simulink model "Model7"  (R2022b)
settings: Solver=VariableStepAuto  StartTime=0.0  StopTime=10.0  RelTol=1e-3
model workspace (MAT data in the model file):
  Freq = Simulink.Parameter
  Freq.Value = 2000000
  Freq.DataType = 'auto'
  Freq.Complexity = 'real'
  Freq.Dimensions = [1 1]
  Freq2 = Simulink.Parameter
  Freq2.Value = 6000000
  Freq2.DataType = 'auto'
  Freq2.Complexity = 'real'
  Freq2.Dimensions = [1 1]
  Freq3 = Simulink.Parameter
  Freq3.Value = 3000000
  Freq3.DataType = 'auto'
  Freq3.Complexity = 'real'
  Freq3.Dimensions = [1 1]
  Freq4 = Simulink.Parameter
  Freq4.Value = 10000000
  Freq4.DataType = 'auto'
  Freq4.Complexity = 'real'
  Freq4.Dimensions = [1 1]
  fsr = 20
libraries: commdigbbndam3 x5, commrandsrc3 x4, dspfdesign x2, commchan3 x1, commsink2 x1, commutil2 x1, simulink x1
settings Model: Creator=Ceribro  LastModifiedBy=Ceribro

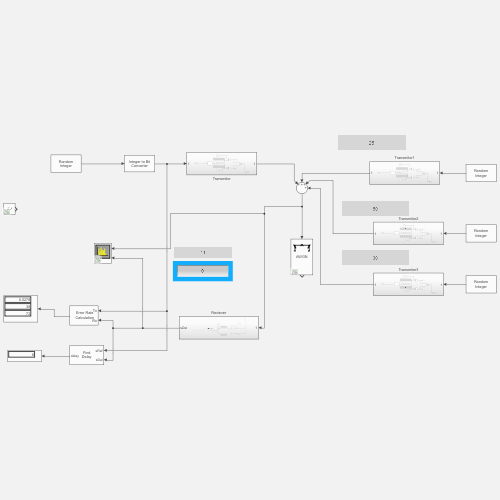
[thumbnail: Simulink's stored preview of the top-level diagram]
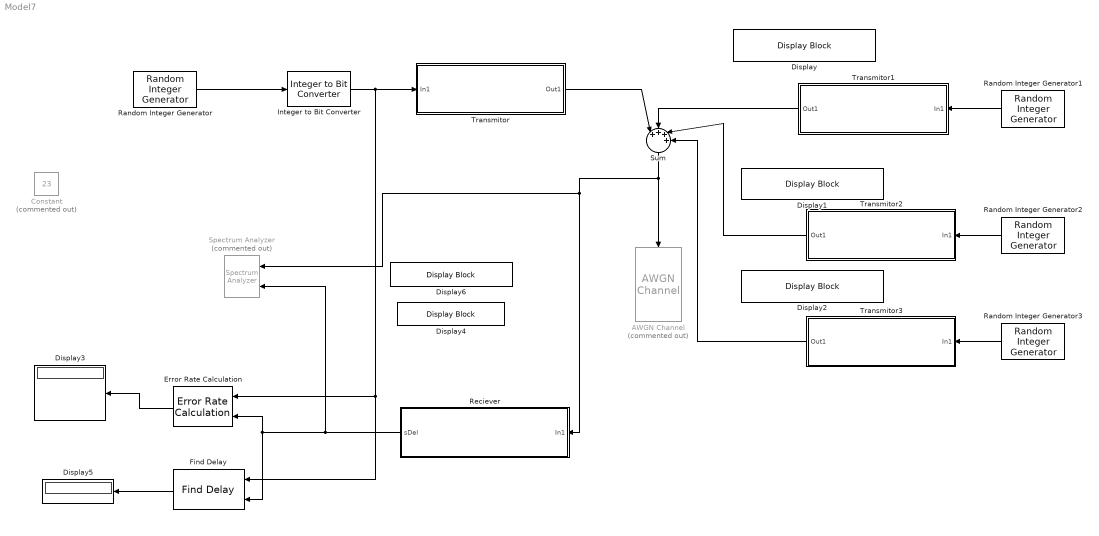
== system Model7 ==
  AWGN Channel : commchan3/AWGN Channel  Commented=on  InputProcessing=Columns as channels (frame based)  seed=67  noiseMode="Signal to noise ratio  (SNR)"  EbNodB=10  EsNodB=10  SNRdB=-10  bitsPerSym=1  Ps=1  Tsym=1  variance=1
  Constant : Constant  Commented=on  Value=23  SampleTime=0.01
  Display{,1..2,4,6} (5 alike) : DisplayBlock  LabelPosition=Hide  Transparency=1
  Display3 : Display
  Display5 : Display
  Error Rate Calculation : commsink2/Error Rate Calculation  N=0  st_delay=0  cp_mode=Entire frame  subframe=[]  PMode=Port  WsName=ErrorVec  RsMode2=off  stop=off  numErr=100  maxBits=1e6
      settings: LibrarySourceBlock=|
      | commhdlsink/Error Rate
      | Calculation
  Find Delay : commutil2/Find Delay  corrLength=10  chgSigOP=off  stopUpdate=off  numConstDelay=3
  Integer to Bit Converter : simulink/Logic and Bit Operations/Integer to Bit Converter  nbits=6  signedInputValues=Unsigned  bitOrder=MSB first  outDtype=Inherit via internal rule
  Random Integer Generator{,1..3} (4 alike) : commrandsrc3/Random Integer Generator  SetSize=64  SeedSource=Auto  Seed=0  SampleTime=0.1  SamplesPerFrame=1  OutputDataType=double  SimulateUsing=Interpreted execution
  Reciever : Subsystem
  Spectrum Analyzer : SpectrumAnalyzer  Commented=on  NumInputPorts=2
  Sum : Sum  Inputs=|++++
  Transmitor : Subsystem
  Transmitor1 : Subsystem
  Transmitor2 : Subsystem
  Transmitor3 : Subsystem
  wires:
  Transmitor/1(Out1) -> Sum/1
  Random Integer Generator/1 -> Integer to Bit Converter/1
  Random Integer Generator1/1 -> Transmitor1/1(In1)
  Sum/1 -> Spectrum Analyzer/1, Reciever/1(In1), AWGN Channel/1
  Transmitor1/1(Out1) -> Sum/2
  Transmitor2/1(Out1) -> Sum/3
  Random Integer Generator2/1 -> Transmitor2/1(In1)
  Random Integer Generator3/1 -> Transmitor3/1(In1)
  Transmitor3/1(Out1) -> Sum/4
  Find Delay/1 -> Display5/1
  Error Rate Calculation/1 -> Display3/1
  Reciever/1(sDel) -> Error Rate Calculation/2, Find Delay/2, Spectrum Analyzer/2
  Integer to Bit Converter/1 -> Find Delay/1, Error Rate Calculation/1, Transmitor/1(In1)

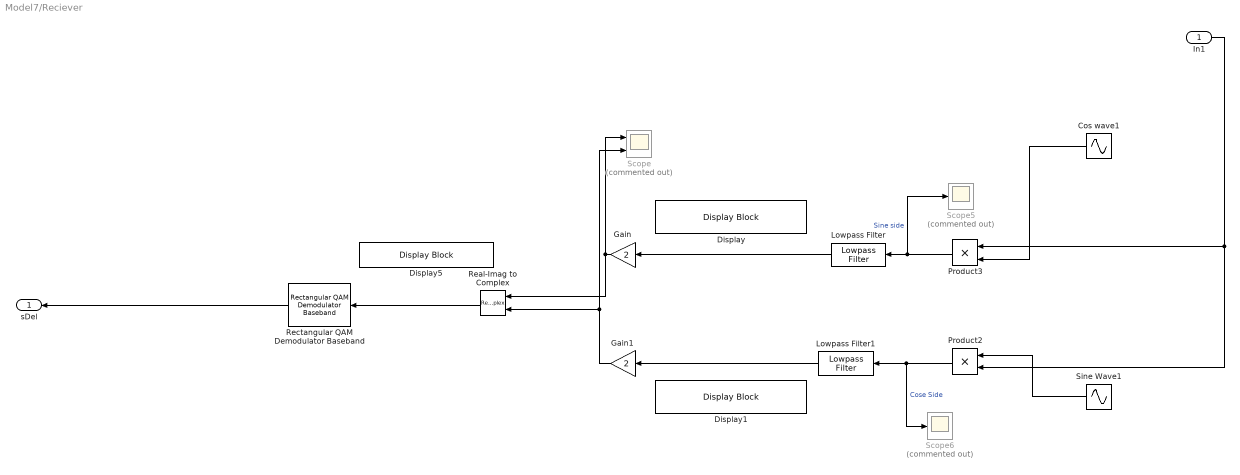
== system Model7/Reciever ==
  In1 : Inport
  Cos wave1 : Sin  Frequency=2*pi*Freq  Phase=pi/2  SampleTime=1/44100  VectorParams1D=off
  Display : DisplayBlock  LabelPosition=Hide  Transparency=1
  Display1 : DisplayBlock  LabelPosition=Hide  Transparency=1
  Display5 : DisplayBlock  LabelPosition=Hide  Transparency=1
  Gain : Gain  Gain=2
  Gain1 : Gain  Gain=2
  Lowpass Filter : dspfdesign/Lowpass Filter  FilterType=FIR  DesignForMinimumOrder=on  FilterOrder=50  PassbandFrequency=0.5e3  StopbandFrequency=1e3  PassbandRipple=0.1  StopbandAttenuation=80  InheritSampleRate=off  SampleRate=44100  SimulateUsing=Interpreted execution  roundingMode=Floor  coeffsDataTypeStr=fixdt(1,16)
  Lowpass Filter1 : dspfdesign/Lowpass Filter  FilterType=FIR  DesignForMinimumOrder=on  FilterOrder=50  PassbandFrequency=0.5e3  StopbandFrequency=1e3  PassbandRipple=0.1  StopbandAttenuation=80  InheritSampleRate=off  SampleRate=44100  SimulateUsing=Interpreted execution  roundingMode=Floor  coeffsDataTypeStr=fixdt(1,16)
  Product2 : Product
  Product3 : Product
  Real-Imag to Complex : RealImagToComplex
  Rectangular QAM Demodulator Baseband : commdigbbndam3/Rectangular QAM Demodulator Baseband  M=64  OutType=Bit  DecType=Hard decision  VarSource=Dialog  Variance=1  Dec=Binary  Mapping=[0:15]  PowType=Min. distance between symbols  MinDist=2  AvgPow=1  PeakPow=1  Ph=0  outDtype1=Inherit via internal rule  outDtype2=Inherit via internal rule  derotateFactorWordLen=16  derotateFactorDataTypeStr=Inherit: Same word length as input  derotateFactorLastDataTypeStr=Inherit: Same word length as input  denormFactorWordLen=16  denormFactorDataTypeStr=Inherit: Same word length as input  denormFactorLastDataTypeStr=Inherit: Same word length as input  prodOutWordLen=32  prodOutOverflowMode=Wrap  prodOutRoundingMode=Floor  prodOutOvFlMode=off  prodOutOvFlModeLastStrValue=off  sumWordLen=32
      settings: LibrarySourceBlock=|
      | commhdldigbbndam/Rectangular QAM
      | Demodulator
      | Baseband
  Scope : Scope  Commented=on  NumInputPorts=2
  Scope5 : Scope  Commented=on
  Scope6 : Scope  Commented=on
  "Sine Wave1 " : Sin  Frequency=2*pi*Freq  SampleTime=1/44100
  sDel : Outport
  wires:
  Cos wave1/1 -> Product3/2
  "Sine Wave1 "/1 -> Product2/1
  Gain/1 -> Scope/1, Real-Imag to Complex/1
  Gain1/1 -> Real-Imag to Complex/2, Scope/2
  Real-Imag to Complex/1 -> Rectangular QAM Demodulator Baseband/1
  Product3/1 -> Lowpass Filter/1, Scope5/1  "Sine side"
  In1/1 -> Product2/2, Product3/1
  Lowpass Filter/1 -> Gain/1
  Product2/1 -> Lowpass Filter1/1, Scope6/1  "Cose Side"
  Lowpass Filter1/1 -> Gain1/1
  Rectangular QAM Demodulator Baseband/1 -> sDel/1

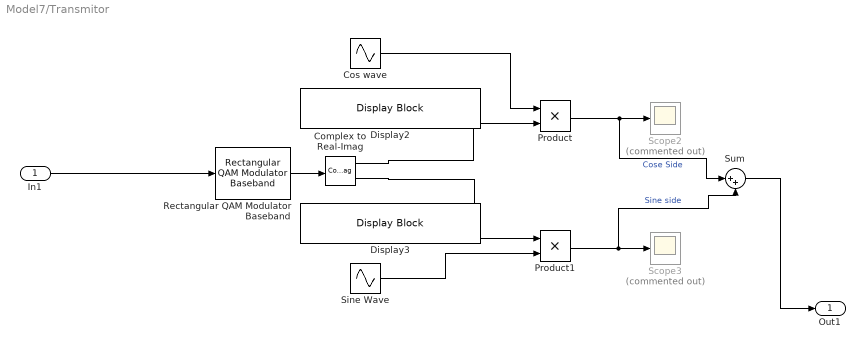
== system Model7/Transmitor ==
  In1 : Inport
  Complex to Real-Imag : ComplexToRealImag
  Cos wave : Sin  Frequency=2*pi*Freq  Phase=pi/2  SampleTime=1/44100  VectorParams1D=off
  Display2 : DisplayBlock  LabelPosition=Hide  Transparency=1
  Display3 : DisplayBlock  LabelPosition=Hide  Transparency=1
  Product : Product
  Product1 : Product
  Rectangular QAM Modulator Baseband : commdigbbndam3/Rectangular QAM Modulator Baseband  M=64  InType=Bit  Enc=Binary  Mapping=[0:15]  PowType=Min. distance between symbols  MinDist=2  AvgPow=1  PeakPow=1  Ph=0  outDtype=Fixed-point  outWordLen=16  outUDDataType=sfix(16)  outFracLenMode=User-defined  outFracLen=0  outDataTypeStr=fixdt(1,16,0)  outLastDataTypeStr=fixdt(1,16,0)
      settings: LibrarySourceBlock=|
      | commhdldigbbndam/Rectangular QAM
      | Modulator
      | Baseband
  Scope2 : Scope  Commented=on
  Scope3 : Scope  Commented=on
  "Sine Wave " : Sin  Frequency=2*pi*Freq  SampleTime=1/44100  VectorParams1D=off
  Sum : Sum  Inputs=|++
  Out1 : Outport
  wires:
  Product/1 -> Scope2/1, Sum/1  "Cose Side"
  Rectangular QAM Modulator Baseband/1 -> Complex to Real-Imag/1
  Product1/1 -> Scope3/1, Sum/2  "Sine side"
  Complex to Real-Imag/1 -> Product/2
  "Sine Wave "/1 -> Product1/2
  Cos wave/1 -> Product/1
  Complex to Real-Imag/2 -> Product1/1
  In1/1 -> Rectangular QAM Modulator Baseband/1
  Sum/1 -> Out1/1

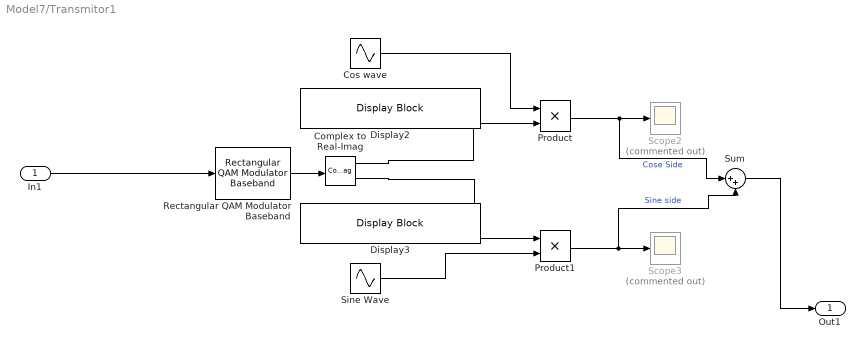
== system Model7/Transmitor1 ==
  In1 : Inport
  Complex to Real-Imag : ComplexToRealImag
  Cos wave : Sin  Frequency=2*pi*Freq2  Phase=pi/2  SampleTime=1/44100  VectorParams1D=off
  Display2 : DisplayBlock  LabelPosition=Hide  Transparency=1
  Display3 : DisplayBlock  LabelPosition=Hide  Transparency=1
  Product : Product
  Product1 : Product
  Rectangular QAM Modulator Baseband : commdigbbndam3/Rectangular QAM Modulator Baseband  M=64  InType=Integer  Enc=Binary  Mapping=[0:15]  PowType=Min. distance between symbols  MinDist=2  AvgPow=1  PeakPow=1  Ph=0  outDtype=Fixed-point  outWordLen=16  outUDDataType=sfix(16)  outFracLenMode=User-defined  outFracLen=0  outDataTypeStr=fixdt(1,16,0)  outLastDataTypeStr=fixdt(1,16,0)
      settings: LibrarySourceBlock=|
      | commhdldigbbndam/Rectangular QAM
      | Modulator
      | Baseband
  Scope2 : Scope  Commented=on
  Scope3 : Scope  Commented=on
  "Sine Wave " : Sin  Frequency=2*pi*Freq2  SampleTime=1/44100  VectorParams1D=off
  Sum : Sum  Inputs=|++
  Out1 : Outport
  wires:
  Product/1 -> Scope2/1, Sum/1  "Cose Side"
  Rectangular QAM Modulator Baseband/1 -> Complex to Real-Imag/1
  Product1/1 -> Scope3/1, Sum/2  "Sine side"
  Complex to Real-Imag/1 -> Product/2
  "Sine Wave "/1 -> Product1/2
  Cos wave/1 -> Product/1
  Complex to Real-Imag/2 -> Product1/1
  In1/1 -> Rectangular QAM Modulator Baseband/1
  Sum/1 -> Out1/1

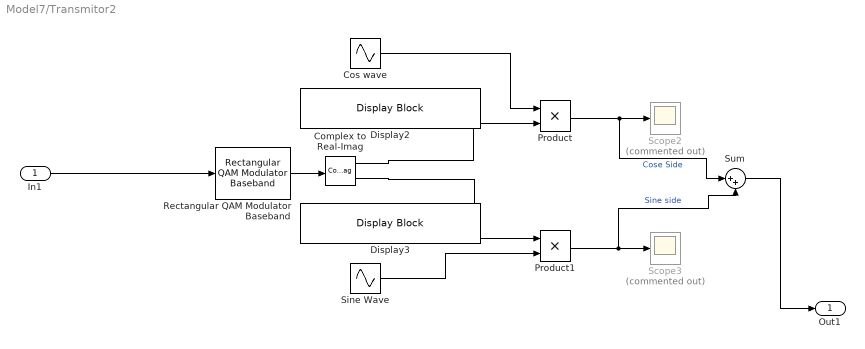
== system Model7/Transmitor2 ==
  In1 : Inport
  Complex to Real-Imag : ComplexToRealImag
  Cos wave : Sin  Frequency=2*pi*Freq3  Phase=pi/2  SampleTime=1/44100  VectorParams1D=off
  Display2 : DisplayBlock  LabelPosition=Hide  Transparency=1
  Display3 : DisplayBlock  LabelPosition=Hide  Transparency=1
  Product : Product
  Product1 : Product
  Rectangular QAM Modulator Baseband : commdigbbndam3/Rectangular QAM Modulator Baseband  M=64  InType=Integer  Enc=Binary  Mapping=[0:15]  PowType=Min. distance between symbols  MinDist=2  AvgPow=1  PeakPow=1  Ph=0  outDtype=Fixed-point  outWordLen=16  outUDDataType=sfix(16)  outFracLenMode=User-defined  outFracLen=0  outDataTypeStr=fixdt(1,16,0)  outLastDataTypeStr=fixdt(1,16,0)
      settings: LibrarySourceBlock=|
      | commhdldigbbndam/Rectangular QAM
      | Modulator
      | Baseband
  Scope2 : Scope  Commented=on
  Scope3 : Scope  Commented=on
  "Sine Wave " : Sin  Frequency=2*pi*Freq3  SampleTime=1/44100  VectorParams1D=off
  Sum : Sum  Inputs=|++
  Out1 : Outport
  wires:
  Product/1 -> Scope2/1, Sum/1  "Cose Side"
  Rectangular QAM Modulator Baseband/1 -> Complex to Real-Imag/1
  Product1/1 -> Scope3/1, Sum/2  "Sine side"
  Complex to Real-Imag/1 -> Product/2
  "Sine Wave "/1 -> Product1/2
  Cos wave/1 -> Product/1
  Complex to Real-Imag/2 -> Product1/1
  In1/1 -> Rectangular QAM Modulator Baseband/1
  Sum/1 -> Out1/1

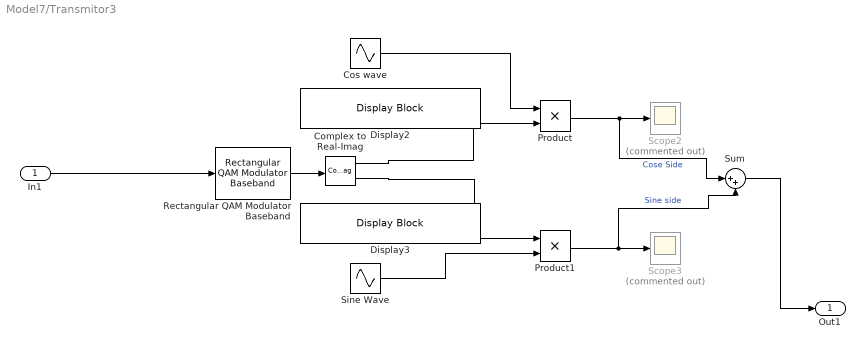
== system Model7/Transmitor3 ==
  In1 : Inport
  Complex to Real-Imag : ComplexToRealImag
  Cos wave : Sin  Frequency=2*pi*Freq4  Phase=pi/2  SampleTime=1/44100  VectorParams1D=off
  Display2 : DisplayBlock  LabelPosition=Hide  Transparency=1
  Display3 : DisplayBlock  LabelPosition=Hide  Transparency=1
  Product : Product
  Product1 : Product
  Rectangular QAM Modulator Baseband : commdigbbndam3/Rectangular QAM Modulator Baseband  M=64  InType=Integer  Enc=Binary  Mapping=[0:15]  PowType=Min. distance between symbols  MinDist=2  AvgPow=1  PeakPow=1  Ph=0  outDtype=Fixed-point  outWordLen=16  outUDDataType=sfix(16)  outFracLenMode=User-defined  outFracLen=0  outDataTypeStr=fixdt(1,16,0)  outLastDataTypeStr=fixdt(1,16,0)
      settings: LibrarySourceBlock=|
      | commhdldigbbndam/Rectangular QAM
      | Modulator
      | Baseband
  Scope2 : Scope  Commented=on
  Scope3 : Scope  Commented=on
  "Sine Wave " : Sin  Frequency=2*pi*Freq4  SampleTime=1/44100  VectorParams1D=off
  Sum : Sum  Inputs=|++
  Out1 : Outport
  wires:
  Product/1 -> Scope2/1, Sum/1  "Cose Side"
  Rectangular QAM Modulator Baseband/1 -> Complex to Real-Imag/1
  Product1/1 -> Scope3/1, Sum/2  "Sine side"
  Complex to Real-Imag/1 -> Product/2
  "Sine Wave "/1 -> Product1/2
  Cos wave/1 -> Product/1
  Complex to Real-Imag/2 -> Product1/1
  In1/1 -> Rectangular QAM Modulator Baseband/1
  Sum/1 -> Out1/1
